simulink model "GuiSetpointHandler"  (R2016b)
settings: Solver=FixedStepAuto  StartTime=0.0  StopTime=10.0  RelTol=1e-3  EnableMultiTasking=on
settings Model: Creator=march  LastModifiedBy=snyke7
settings SolverCC: EnableConcurrentExecution=on
settings DataIOCC: SaveFormat=StructureWithTime
settings OptimizationCC: BlockReduction=off  OptimizeBlockIOStorage=off  BufferReuse=off  GlobalBufferReuse=off  ExpressionFolding=off  LocalBlockOutputs=off
settings HardwareCC: ProdBitPerPointer=32  ProdBitPerSizeT=32  ProdBitPerPtrDiffT=32  ProdLargestAtomicFloat=None  ProdWordSize=32  ProdLongLongMode=on  ProdHWDeviceType=Generic->32-bit x86 compatible
settings RTWCC: SystemTargetFile=slrt.tlc  TemplateMakefile=slrt_default_tmf  Description=Simulink Real-Time  RTWCompilerOptimization=on
settings TargetCC: CodeReplacementLibrary=XPC_BLAS  ParMdlRefBuildCompliant=on  ConcurrentExecutionCompliant=on  GeneratePreprocessorConditionals=Use local settings  MatFileLogging=on  MATLABClassNameForMDSCustomization=xpcAperiodicCustomization

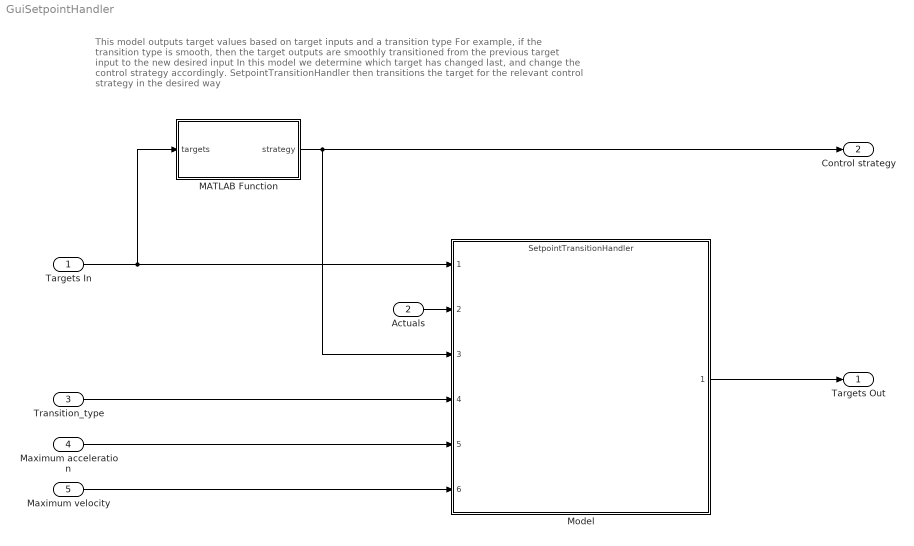
== system GuiSetpointHandler ==
  note: This model outputs target values based on target inputs and a transition type
      | For example, if the transition type is smooth, then the target outputs are smoothly transitioned from the previous target input to the new desired input
      |
      | In this model we determine which target has changed last, and change the control strategy accordingly. SetpointTransitionHandler then transitions the target for the relevant control strategy in the desired way
  Targets In : Inport
  Actuals : Inport  Port=2  PortDimensions=[ 3 1 ]
  Transition_type : Inport  Port=3
  Maximum acceleration : Inport  Port=4
  Maximum velocity : Inport  Port=5
  MATLAB Function : MATLAB Function  TreatAsAtomicUnit=on
  Model : ModelReference  ModelNameDialog=SetpointTransitionHandler  SimulationMode=Normal  ModelReferenceVersion=1.43
  Targets Out : Outport
  Control strategy : Outport  Port=2  OutDataTypeStr=Enum: ControlStrategy
  wires:
  Targets In/1 -> Model/1, MATLAB Function/1(targets)
  MATLAB Function/1(strategy) -> Model/3, Control strategy/1
  Actuals/1 -> Model/2
  Transition_type/1 -> Model/4
  Maximum acceleration/1 -> Model/5
  Maximum velocity/1 -> Model/6
  Model/1 -> Targets Out/1

== matlab function GuiSetpointHandler/MATLAB Function ==
  data: targets input size=[ 3 1 ]; strategy output Enum: ControlStrategy
function strategy = getLastChanged(targets)
persistent lastTargets;
persistent lastStrategy;
if isempty(lastTargets)
    lastTargets = [0;0;0];
    lastStrategy = ControlStrategy.torque;
end
% initialize strategy
% finds the first index that changed
firstChangedIndex = find(lastTargets ~= targets,1);
if isempty(firstChangedIndex)
    strategy = lastStrategy;
else
    strategy = ControlStrategy(firstChangedIndex(1));
end
lastStrategy = strategy;
lastTargets = targets;
end
